simulink model "ThdRwLtStFwdBkwdIsPosChk"  (R2018b)
settings: Solver=FixedStepDiscrete  StartTime=0.0  StopTime=10.0  FixedStep=0.01  RelTol=1e-3
undefined symbols (not defined in the file or in its folder): KeSMSuThirdRwStFwdBkwdPosDelta_Val, KeSMSuThirdRwStFwdBkwdPosTolr_Val, KeSMSuVehicleModelConfig_Val
libraries: StIsPosChkLib x17, simulink x5
(part 1 of 2)
settings Model: Creator=sn2xws  LastModifiedBy=sn55gm
settings Model: ModifiedHistory=|
  | 2024.3.14
  | V2.3.0
  | Bug 813950 童锁Lock，Mode1_Easy Entry Mode 不应调用失败
  | 2024.7.5 V3.0.0 557模式流程V1.9
  | 2024.8.28 V3.0.1 Lug模式修改干涉判断成功的逻辑
  | 2024.9.6 V3.0.2 新增Md56，注释不用的模式
  | 2024.10.14 V3.0.3 新增Md57 Md58
  | 2024.10.28 V3.0.4 6s版本不选md12目标位置
  | 2024.11.11 V3.0.5 vip 判断成功不看三排
  | 2024.12.24 V3.0.6 CR 960542 7S智享退出模式左右同时调用时，三排座椅前后使用逻辑变更
  | 2025.2.19 V3.8.0 Bug 991386 Md1 三排占座时未移动且报了成功
  | 25.7.1 V3.13.0 新增Md61 Md62
  | 25.7.17 V3.13.1 BUG 1089114
  | 25.8.12 V3.13.2 BUG 1109205
settings DataIOCC: SaveFormat=StructureWithTime
settings OptimizationCC: DefaultParameterBehavior=Inlined  EnhancedBackFolding=on  PassReuseOutputArgsAs=Individual arguments  ZeroExternalMemoryAtStartup=off  ZeroInternalMemoryAtStartup=off  OptimizeBlockOrder=speed  DifferentSizesBufferReuse=on  OptimizationCustomize=off
settings DebuggingCC: ParameterTunabilityLossMsg=error
settings ModelReferenceCC: ModelReferenceNumInstancesAllowed=Single
settings SFSimCC: MATLABDynamicMemAlloc=off
settings RTWCC: SystemTargetFile=autosar.tlc  GenCodeOnly=on  TemplateMakefile=ert_default_tmf  Description=AUTOSAR  GenerateReport=on  IncludeHyperlinkInReport=on  LaunchReport=on  GenerateTraceInfo=on  GenerateTraceReport=on  GenerateTraceReportSl=on  GenerateTraceReportSf=on  GenerateTraceReportEml=on
settings CodeAppCC: ForceParamTrailComments=on  IgnoreCustomStorageClasses=off  OperatorAnnotations=on  SimulinkDataObjDesc=on  SFDataObjDesc=on  InsertBlockDesc=on
settings STFCustomTargetCC: TargetLangStandard=C99 (ISO)  MultiwordLength=256  ParMdlRefBuildCompliant=on  CompOptLevelCompliant=on  IncludeMdlTerminateFcn=off  CombineOutputUpdateFcns=on  SuppressErrorStatus=on  ERTCustomFileBanners=on  SupportNonFinite=off  SupportComplex=off  SupportContinuousTime=off  SupportNonInlinedSFcns=off  RemoveResetFunc=on  MATLABClassNameForMDSCustomization=Simulink.SoftwareTarget.ERTCustomization  AutosarCompliant=on  UseToolchainInfoCompliant=on  LookupTableObjectStructAxisOrder=2,1,3,4,...  LUTObjectStructOrderEvenSpacing=Size,Table,Breakpoints  SystemTargetFile=autosar.tlc
settings ERTTargetCC: TargetLangStandard=C99 (ISO)  ConcurrentExecutionCompliant=off  IncludeMdlTerminateFcn=off  SuppressErrorStatus=on  SupportNonFinite=off  SupportComplex=off  ModelStepFunctionPrototypeControlCompliant=off  CPPClassGenCompliant=off  AutosarCompliant=on  LookupTableObjectStructAxisOrder=2,1,3,4,...  LUTObjectStructOrderEvenSpacing=Size,Table,Breakpoints  InlinedParameterPlacement=NonHierarchical  ERTCustomFileTemplate=example_file_process.tlc  ERTFilePackagingFormat=Compact

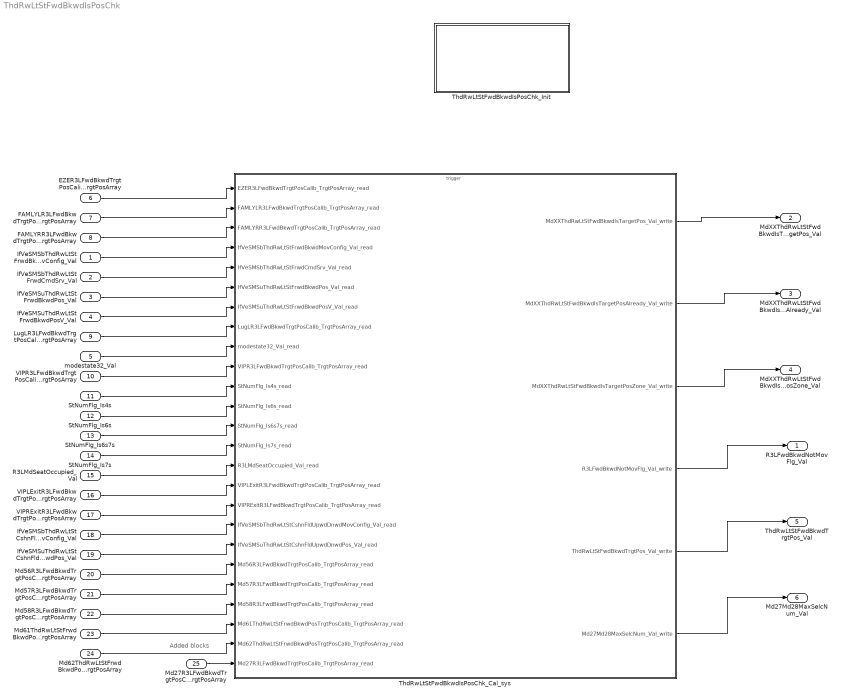
== system ThdRwLtStFwdBkwdIsPosChk ==
  note: Added blocks
  IfVeSMSbThdRwLtStFrwdBkwdMovConfig_Val : Inport  OutDataTypeStr=boolean  PortDimensions=1
  IfVeSMSbThdRwLtStFrwdCmdSrv_Val : Inport  Port=2  OutDataTypeStr=boolean  PortDimensions=1
  IfVeSMSuThdRwLtStFrwdBkwdPos_Val : Inport  Port=3  OutDataTypeStr=uint16  PortDimensions=1
  IfVeSMSuThdRwLtStFrwdBkwdPosV_Val : Inport  Port=4  OutDataTypeStr=boolean  PortDimensions=1
  modestate32_Val : Inport  Port=5  OutDataTypeStr=uint32  PortDimensions=1
  EZER3LFwdBkwdTrgtPosCalib_TrgtPosArray : Inport  Description=|  Port=6  OutDataTypeStr=uint16  PortDimensions=3
      | 0:Pos
      | 1:Max
      | 2:Min
  FAMLYLR3LFwdBkwdTrgtPosCalib_TrgtPosArray : Inport  Description=|  Port=7  OutDataTypeStr=uint16  PortDimensions=3
      | 0:Pos
      | 1:Max
      | 2:Min
  FAMLYRR3LFwdBkwdTrgtPosCalib_TrgtPosArray : Inport  Description=|  Port=8  OutDataTypeStr=uint16  PortDimensions=3
      | 0:Pos
      | 1:Max
      | 2:Min
  LugLR3LFwdBkwdTrgtPosCalib_TrgtPosArray : Inport  Description=|  Port=9  OutDataTypeStr=uint16  PortDimensions=3
      | 0:Pos
      | 1:Max
      | 2:Min
  VIPR3LFwdBkwdTrgtPosCalib_TrgtPosArray : Inport  Description=|  Port=10  OutDataTypeStr=uint16  PortDimensions=3
      | 0:Pos
      | 1:Max
      | 2:Min
  StNumFlg_Is4s : Inport  Port=11  OutDataTypeStr=boolean  PortDimensions=1
  StNumFlg_Is6s : Inport  Port=12  OutDataTypeStr=boolean  PortDimensions=1
  StNumFlg_Is6s7s : Inport  Port=13  OutDataTypeStr=boolean  PortDimensions=1
  StNumFlg_Is7s : Inport  Port=14  OutDataTypeStr=boolean  PortDimensions=1
  R3LMdSeatOccupied_Val : Inport  Port=15  OutDataTypeStr=boolean  PortDimensions=1
  VIPLExitR3LFwdBkwdTrgtPosCalib_TrgtPosArray : Inport  Description=|  Port=16  OutDataTypeStr=uint16  PortDimensions=3
      | 0:Pos
      | 1:Max
      | 2:Min
  VIPRExitR3LFwdBkwdTrgtPosCalib_TrgtPosArray : Inport  Description=|  Port=17  OutDataTypeStr=uint16  PortDimensions=3
      | 0:Pos
      | 1:Max
      | 2:Min
  IfVeSMSbThdRwLtStCshnFldUpwdDnwdMovConfig_Val : Inport  Port=18  OutDataTypeStr=boolean  PortDimensions=1
  IfVeSMSuThdRwLtStCshnFldUpwdDnwdPos_Val : Inport  Port=19  OutDataTypeStr=uint16  PortDimensions=1
  Md56R3LFwdBkwdTrgtPosCalib_TrgtPosArray : Inport  Description=|  Port=20  OutDataTypeStr=uint16  PortDimensions=3
      | 0:Pos
      | 1:Max
      | 2:Min
  Md57R3LFwdBkwdTrgtPosCalib_TrgtPosArray : Inport  Description=|  Port=21  OutDataTypeStr=uint16  PortDimensions=3
      | 0:Pos
      | 1:Max
      | 2:Min
  Md58R3LFwdBkwdTrgtPosCalib_TrgtPosArray : Inport  Description=|  Port=22  OutDataTypeStr=uint16  PortDimensions=3
      | 0:Pos
      | 1:Max
      | 2:Min
  Md61ThdRwLtStFrwdBkwdPosTrgtPosCalib_TrgtPosArray : Inport  Description=|  Port=23  OutDataTypeStr=uint16  PortDimensions=3
      | 0:Pos
      | 1:Max
      | 2:Min
  Md62ThdRwLtStFrwdBkwdPosTrgtPosCalib_TrgtPosArray : Inport  Description=|  Port=24  OutDataTypeStr=uint16  PortDimensions=3
      | 0:Pos
      | 1:Max
      | 2:Min
  Md27R3LFwdBkwdTrgtPosCalib_TrgtPosArray : Inport  Description=|  Port=25  OutDataTypeStr=uint16  PortDimensions=3
      | 0:Pos
      | 1:Max
      | 2:Min
  ThdRwLtStFwdBkwdIsPosChk_Cal_sys : Subsystem
  ThdRwLtStFwdBkwdIsPosChk_Init : Subsystem
  R3LFwdBkwdNotMovFlg_Val : Outport  OutDataTypeStr=boolean  PortDimensions=1
  MdXXThdRwLtStFwdBkwdIsTargetPos_Val : Outport  Port=2  OutDataTypeStr=uint32  PortDimensions=1
  MdXXThdRwLtStFwdBkwdIsTargetPosAlready_Val : Outport  Port=3  OutDataTypeStr=uint32  PortDimensions=1
  MdXXThdRwLtStFwdBkwdIsTargetPosZone_Val : Outport  Port=4  OutDataTypeStr=uint32  PortDimensions=1
  ThdRwLtStFwdBkwdTrgtPos_Val : Outport  Port=5  OutDataTypeStr=uint16  PortDimensions=1
  Md27Md28MaxSelcNum_Val : Outport  Port=6  OutDataTypeStr=uint8  PortDimensions=1
  wires:
  ThdRwLtStFwdBkwdIsPosChk_Cal_sys/1(MdXXThdRwLtStFwdBkwdIsTargetPos_Val_write) -> MdXXThdRwLtStFwdBkwdIsTargetPos_Val/1
  ThdRwLtStFwdBkwdIsPosChk_Cal_sys/2(MdXXThdRwLtStFwdBkwdIsTargetPosAlready_Val_write) -> MdXXThdRwLtStFwdBkwdIsTargetPosAlready_Val/1
  ThdRwLtStFwdBkwdIsPosChk_Cal_sys/3(MdXXThdRwLtStFwdBkwdIsTargetPosZone_Val_write) -> MdXXThdRwLtStFwdBkwdIsTargetPosZone_Val/1
  ThdRwLtStFwdBkwdIsPosChk_Cal_sys/4(R3LFwdBkwdNotMovFlg_Val_write) -> R3LFwdBkwdNotMovFlg_Val/1
  ThdRwLtStFwdBkwdIsPosChk_Cal_sys/5(ThdRwLtStFwdBkwdTrgtPos_Val_write) -> ThdRwLtStFwdBkwdTrgtPos_Val/1
  EZER3LFwdBkwdTrgtPosCalib_TrgtPosArray/1 -> ThdRwLtStFwdBkwdIsPosChk_Cal_sys/1(EZER3LFwdBkwdTrgtPosCalib_TrgtPosArray_read)
  FAMLYLR3LFwdBkwdTrgtPosCalib_TrgtPosArray/1 -> ThdRwLtStFwdBkwdIsPosChk_Cal_sys/2(FAMLYLR3LFwdBkwdTrgtPosCalib_TrgtPosArray_read)
  FAMLYRR3LFwdBkwdTrgtPosCalib_TrgtPosArray/1 -> ThdRwLtStFwdBkwdIsPosChk_Cal_sys/3(FAMLYRR3LFwdBkwdTrgtPosCalib_TrgtPosArray_read)
  IfVeSMSbThdRwLtStFrwdBkwdMovConfig_Val/1 -> ThdRwLtStFwdBkwdIsPosChk_Cal_sys/4(IfVeSMSbThdRwLtStFrwdBkwdMovConfig_Val_read)
  IfVeSMSbThdRwLtStFrwdCmdSrv_Val/1 -> ThdRwLtStFwdBkwdIsPosChk_Cal_sys/5(IfVeSMSbThdRwLtStFrwdCmdSrv_Val_read)
  IfVeSMSuThdRwLtStFrwdBkwdPos_Val/1 -> ThdRwLtStFwdBkwdIsPosChk_Cal_sys/6(IfVeSMSuThdRwLtStFrwdBkwdPos_Val_read)
  IfVeSMSuThdRwLtStFrwdBkwdPosV_Val/1 -> ThdRwLtStFwdBkwdIsPosChk_Cal_sys/7(IfVeSMSuThdRwLtStFrwdBkwdPosV_Val_read)
  LugLR3LFwdBkwdTrgtPosCalib_TrgtPosArray/1 -> ThdRwLtStFwdBkwdIsPosChk_Cal_sys/8(LugLR3LFwdBkwdTrgtPosCalib_TrgtPosArray_read)
  modestate32_Val/1 -> ThdRwLtStFwdBkwdIsPosChk_Cal_sys/9(modestate32_Val_read)
  VIPR3LFwdBkwdTrgtPosCalib_TrgtPosArray/1 -> ThdRwLtStFwdBkwdIsPosChk_Cal_sys/10(VIPR3LFwdBkwdTrgtPosCalib_TrgtPosArray_read)
  StNumFlg_Is4s/1 -> ThdRwLtStFwdBkwdIsPosChk_Cal_sys/11(StNumFlg_Is4s_read)
  StNumFlg_Is6s/1 -> ThdRwLtStFwdBkwdIsPosChk_Cal_sys/12(StNumFlg_Is6s_read)
  StNumFlg_Is6s7s/1 -> ThdRwLtStFwdBkwdIsPosChk_Cal_sys/13(StNumFlg_Is6s7s_read)
  StNumFlg_Is7s/1 -> ThdRwLtStFwdBkwdIsPosChk_Cal_sys/14(StNumFlg_Is7s_read)
  R3LMdSeatOccupied_Val/1 -> ThdRwLtStFwdBkwdIsPosChk_Cal_sys/15(R3LMdSeatOccupied_Val_read)
  VIPLExitR3LFwdBkwdTrgtPosCalib_TrgtPosArray/1 -> ThdRwLtStFwdBkwdIsPosChk_Cal_sys/16(VIPLExitR3LFwdBkwdTrgtPosCalib_TrgtPosArray_read)
  VIPRExitR3LFwdBkwdTrgtPosCalib_TrgtPosArray/1 -> ThdRwLtStFwdBkwdIsPosChk_Cal_sys/17(VIPRExitR3LFwdBkwdTrgtPosCalib_TrgtPosArray_read)
  IfVeSMSbThdRwLtStCshnFldUpwdDnwdMovConfig_Val/1 -> ThdRwLtStFwdBkwdIsPosChk_Cal_sys/18(IfVeSMSbThdRwLtStCshnFldUpwdDnwdMovConfig_Val_read)
  IfVeSMSuThdRwLtStCshnFldUpwdDnwdPos_Val/1 -> ThdRwLtStFwdBkwdIsPosChk_Cal_sys/19(IfVeSMSuThdRwLtStCshnFldUpwdDnwdPos_Val_read)
  Md56R3LFwdBkwdTrgtPosCalib_TrgtPosArray/1 -> ThdRwLtStFwdBkwdIsPosChk_Cal_sys/20(Md56R3LFwdBkwdTrgtPosCalib_TrgtPosArray_read)
  Md57R3LFwdBkwdTrgtPosCalib_TrgtPosArray/1 -> ThdRwLtStFwdBkwdIsPosChk_Cal_sys/21(Md57R3LFwdBkwdTrgtPosCalib_TrgtPosArray_read)
  Md58R3LFwdBkwdTrgtPosCalib_TrgtPosArray/1 -> ThdRwLtStFwdBkwdIsPosChk_Cal_sys/22(Md58R3LFwdBkwdTrgtPosCalib_TrgtPosArray_read)
  ThdRwLtStFwdBkwdIsPosChk_Cal_sys/6(Md27Md28MaxSelcNum_Val_write) -> Md27Md28MaxSelcNum_Val/1
  Md61ThdRwLtStFrwdBkwdPosTrgtPosCalib_TrgtPosArray/1 -> ThdRwLtStFwdBkwdIsPosChk_Cal_sys/23(Md61ThdRwLtStFrwdBkwdPosTrgtPosCalib_TrgtPosArray_read)
  Md62ThdRwLtStFrwdBkwdPosTrgtPosCalib_TrgtPosArray/1 -> ThdRwLtStFwdBkwdIsPosChk_Cal_sys/24(Md62ThdRwLtStFrwdBkwdPosTrgtPosCalib_TrgtPosArray_read)
  Md27R3LFwdBkwdTrgtPosCalib_TrgtPosArray/1 -> ThdRwLtStFwdBkwdIsPosChk_Cal_sys/25(Md27R3LFwdBkwdTrgtPosCalib_TrgtPosArray_read)

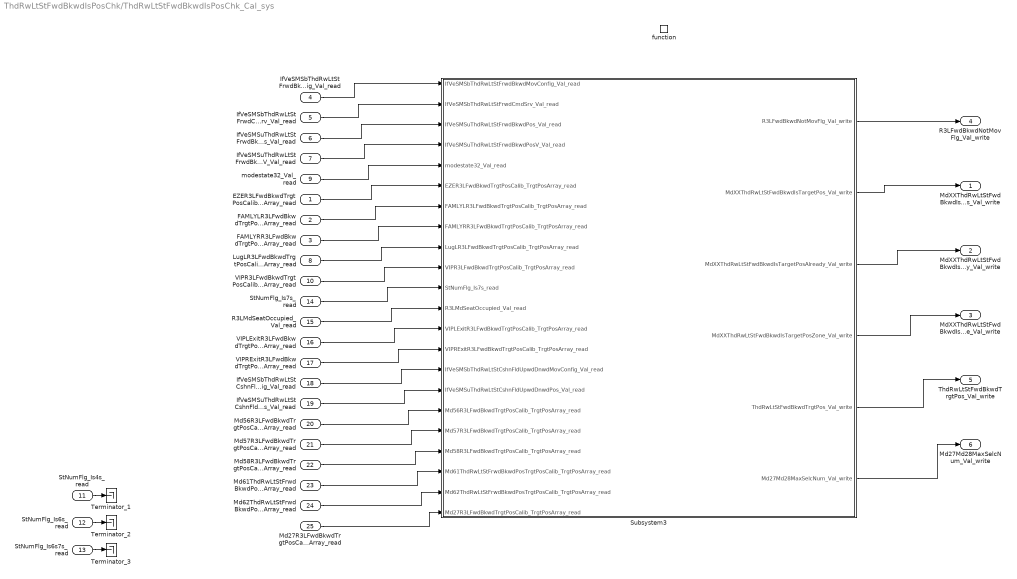
== system ThdRwLtStFwdBkwdIsPosChk/ThdRwLtStFwdBkwdIsPosChk_Cal_sys ==
  EZER3LFwdBkwdTrgtPosCalib_TrgtPosArray_read : Inport
  FAMLYLR3LFwdBkwdTrgtPosCalib_TrgtPosArray_read : Inport  Port=2
  FAMLYRR3LFwdBkwdTrgtPosCalib_TrgtPosArray_read : Inport  Port=3
  IfVeSMSbThdRwLtStFrwdBkwdMovConfig_Val_read : Inport  Port=4
  IfVeSMSbThdRwLtStFrwdCmdSrv_Val_read : Inport  Port=5
  IfVeSMSuThdRwLtStFrwdBkwdPos_Val_read : Inport  Port=6
  IfVeSMSuThdRwLtStFrwdBkwdPosV_Val_read : Inport  Port=7
  LugLR3LFwdBkwdTrgtPosCalib_TrgtPosArray_read : Inport  Port=8
  modestate32_Val_read : Inport  Port=9
  VIPR3LFwdBkwdTrgtPosCalib_TrgtPosArray_read : Inport  Port=10
  StNumFlg_Is4s_read : Inport  Port=11
  StNumFlg_Is6s_read : Inport  Port=12
  StNumFlg_Is6s7s_read : Inport  Port=13
  StNumFlg_Is7s_read : Inport  Port=14
  R3LMdSeatOccupied_Val_read : Inport  Port=15
  VIPLExitR3LFwdBkwdTrgtPosCalib_TrgtPosArray_read : Inport  Port=16
  VIPRExitR3LFwdBkwdTrgtPosCalib_TrgtPosArray_read : Inport  Port=17
  IfVeSMSbThdRwLtStCshnFldUpwdDnwdMovConfig_Val_read : Inport  Port=18
  IfVeSMSuThdRwLtStCshnFldUpwdDnwdPos_Val_read : Inport  Port=19
  Md56R3LFwdBkwdTrgtPosCalib_TrgtPosArray_read : Inport  Port=20
  Md57R3LFwdBkwdTrgtPosCalib_TrgtPosArray_read : Inport  Port=21
  Md58R3LFwdBkwdTrgtPosCalib_TrgtPosArray_read : Inport  Port=22
  Md61ThdRwLtStFrwdBkwdPosTrgtPosCalib_TrgtPosArray_read : Inport  Port=23
  Md62ThdRwLtStFrwdBkwdPosTrgtPosCalib_TrgtPosArray_read : Inport  Port=24
  Md27R3LFwdBkwdTrgtPosCalib_TrgtPosArray_read : Inport  Port=25
  function : TriggerPort  TriggerType=function-call  IsSimulinkFunction=on  FunctionName=ThdRwLtStFwdBkwdIsPosChk_Cal  VariantControl=(inherit)
  Subsystem3 : Subsystem
  Terminator_1 : Terminator
  Terminator_2 : Terminator
  Terminator_3 : Terminator
  MdXXThdRwLtStFwdBkwdIsTargetPos_Val_write : Outport
      settings: EnsureOutportIsVirtual=on
  MdXXThdRwLtStFwdBkwdIsTargetPosAlready_Val_write : Outport  Port=2
      settings: EnsureOutportIsVirtual=on
  MdXXThdRwLtStFwdBkwdIsTargetPosZone_Val_write : Outport  Port=3
      settings: EnsureOutportIsVirtual=on
  R3LFwdBkwdNotMovFlg_Val_write : Outport  Port=4
      settings: EnsureOutportIsVirtual=on
  ThdRwLtStFwdBkwdTrgtPos_Val_write : Outport  Port=5
      settings: EnsureOutportIsVirtual=on
  Md27Md28MaxSelcNum_Val_write : Outport  Port=6
      settings: EnsureOutportIsVirtual=on
  wires:
  Subsystem3/1(R3LFwdBkwdNotMovFlg_Val_write) -> R3LFwdBkwdNotMovFlg_Val_write/1
  Subsystem3/2(MdXXThdRwLtStFwdBkwdIsTargetPos_Val_write) -> MdXXThdRwLtStFwdBkwdIsTargetPos_Val_write/1
  Subsystem3/3(MdXXThdRwLtStFwdBkwdIsTargetPosAlready_Val_write) -> MdXXThdRwLtStFwdBkwdIsTargetPosAlready_Val_write/1
  Subsystem3/4(MdXXThdRwLtStFwdBkwdIsTargetPosZone_Val_write) -> MdXXThdRwLtStFwdBkwdIsTargetPosZone_Val_write/1
  Subsystem3/5(ThdRwLtStFwdBkwdTrgtPos_Val_write) -> ThdRwLtStFwdBkwdTrgtPos_Val_write/1
  IfVeSMSbThdRwLtStFrwdBkwdMovConfig_Val_read/1 -> Subsystem3/1(IfVeSMSbThdRwLtStFrwdBkwdMovConfig_Val_read)
  IfVeSMSbThdRwLtStFrwdCmdSrv_Val_read/1 -> Subsystem3/2(IfVeSMSbThdRwLtStFrwdCmdSrv_Val_read)
  IfVeSMSuThdRwLtStFrwdBkwdPos_Val_read/1 -> Subsystem3/3(IfVeSMSuThdRwLtStFrwdBkwdPos_Val_read)
  IfVeSMSuThdRwLtStFrwdBkwdPosV_Val_read/1 -> Subsystem3/4(IfVeSMSuThdRwLtStFrwdBkwdPosV_Val_read)
  modestate32_Val_read/1 -> Subsystem3/5(modestate32_Val_read)
  EZER3LFwdBkwdTrgtPosCalib_TrgtPosArray_read/1 -> Subsystem3/6(EZER3LFwdBkwdTrgtPosCalib_TrgtPosArray_read)
  FAMLYLR3LFwdBkwdTrgtPosCalib_TrgtPosArray_read/1 -> Subsystem3/7(FAMLYLR3LFwdBkwdTrgtPosCalib_TrgtPosArray_read)
  FAMLYRR3LFwdBkwdTrgtPosCalib_TrgtPosArray_read/1 -> Subsystem3/8(FAMLYRR3LFwdBkwdTrgtPosCalib_TrgtPosArray_read)
  LugLR3LFwdBkwdTrgtPosCalib_TrgtPosArray_read/1 -> Subsystem3/9(LugLR3LFwdBkwdTrgtPosCalib_TrgtPosArray_read)
  VIPR3LFwdBkwdTrgtPosCalib_TrgtPosArray_read/1 -> Subsystem3/10(VIPR3LFwdBkwdTrgtPosCalib_TrgtPosArray_read)
  StNumFlg_Is4s_read/1 -> Terminator_1/1
  StNumFlg_Is6s_read/1 -> Terminator_2/1
  StNumFlg_Is6s7s_read/1 -> Terminator_3/1
  StNumFlg_Is7s_read/1 -> Subsystem3/11(StNumFlg_Is7s_read)
  R3LMdSeatOccupied_Val_read/1 -> Subsystem3/12(R3LMdSeatOccupied_Val_read)
  VIPLExitR3LFwdBkwdTrgtPosCalib_TrgtPosArray_read/1 -> Subsystem3/13(VIPLExitR3LFwdBkwdTrgtPosCalib_TrgtPosArray_read)
  VIPRExitR3LFwdBkwdTrgtPosCalib_TrgtPosArray_read/1 -> Subsystem3/14(VIPRExitR3LFwdBkwdTrgtPosCalib_TrgtPosArray_read)
  IfVeSMSbThdRwLtStCshnFldUpwdDnwdMovConfig_Val_read/1 -> Subsystem3/15(IfVeSMSbThdRwLtStCshnFldUpwdDnwdMovConfig_Val_read)
  IfVeSMSuThdRwLtStCshnFldUpwdDnwdPos_Val_read/1 -> Subsystem3/16(IfVeSMSuThdRwLtStCshnFldUpwdDnwdPos_Val_read)
  Md56R3LFwdBkwdTrgtPosCalib_TrgtPosArray_read/1 -> Subsystem3/17(Md56R3LFwdBkwdTrgtPosCalib_TrgtPosArray_read)
  Md57R3LFwdBkwdTrgtPosCalib_TrgtPosArray_read/1 -> Subsystem3/18(Md57R3LFwdBkwdTrgtPosCalib_TrgtPosArray_read)
  Md58R3LFwdBkwdTrgtPosCalib_TrgtPosArray_read/1 -> Subsystem3/19(Md58R3LFwdBkwdTrgtPosCalib_TrgtPosArray_read)
  Subsystem3/6(Md27Md28MaxSelcNum_Val_write) -> Md27Md28MaxSelcNum_Val_write/1
  Md61ThdRwLtStFrwdBkwdPosTrgtPosCalib_TrgtPosArray_read/1 -> Subsystem3/20(Md61ThdRwLtStFrwdBkwdPosTrgtPosCalib_TrgtPosArray_read)
  Md62ThdRwLtStFrwdBkwdPosTrgtPosCalib_TrgtPosArray_read/1 -> Subsystem3/21(Md62ThdRwLtStFrwdBkwdPosTrgtPosCalib_TrgtPosArray_read)
  ? -> ?
  Md27R3LFwdBkwdTrgtPosCalib_TrgtPosArray_read/1 -> Subsystem3/22(Md27R3LFwdBkwdTrgtPosCalib_TrgtPosArray_read)

== system ThdRwLtStFwdBkwdIsPosChk/ThdRwLtStFwdBkwdIsPosChk_Init ==
  note: Added blocks
  note: Added blocks
  note: Added blocks
  Event Listener : EventListener  EventName=reset
  PA_KeSMSuThirdRwStFwdBkwdPosDelta_Val : Constant  Value=KeSMSuThirdRwStFwdBkwdPosDelta_Val
  PA_KeSMSuThirdRwStFwdBkwdPosTolr_Val : Constant  Value=KeSMSuThirdRwStFwdBkwdPosTolr_Val
  PA_KeSMSuVehicleModelConfig_Val : Constant  Value=KeSMSuVehicleModelConfig_Val
  Terminator_1 : Terminator
  Terminator_2 : Terminator
  Terminator_3 : Terminator
  wires:
  PA_KeSMSuThirdRwStFwdBkwdPosDelta_Val/1 -> Terminator_1/1
  PA_KeSMSuThirdRwStFwdBkwdPosTolr_Val/1 -> Terminator_2/1
  PA_KeSMSuVehicleModelConfig_Val/1 -> Terminator_3/1

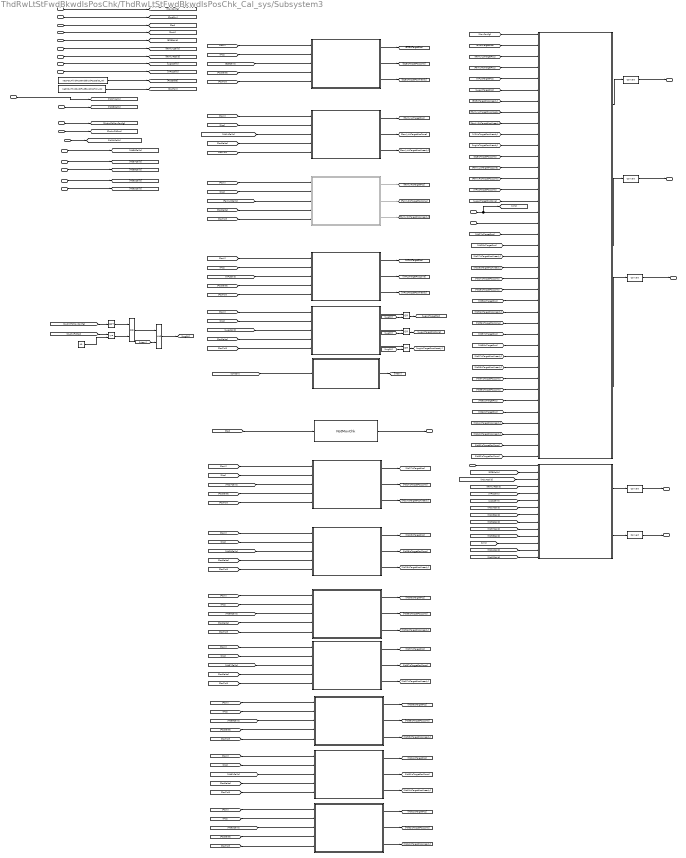
== system ThdRwLtStFwdBkwdIsPosChk/ThdRwLtStFwdBkwdIsPosChk_Cal_sys/Subsystem3 ==
  note: 增加逻辑Lug模式非干涉但是到最前了算成功
  IfVeSMSbThdRwLtStFrwdBkwdMovConfig_Val_read : Inport
  IfVeSMSbThdRwLtStFrwdCmdSrv_Val_read : Inport  Port=2
  IfVeSMSuThdRwLtStFrwdBkwdPos_Val_read : Inport  Port=3
  IfVeSMSuThdRwLtStFrwdBkwdPosV_Val_read : Inport  Port=4
  modestate32_Val_read : Inport  Port=5
  EZER3LFwdBkwdTrgtPosCalib_TrgtPosArray_read : Inport  Port=6
  FAMLYLR3LFwdBkwdTrgtPosCalib_TrgtPosArray_read : Inport  Port=7
  FAMLYRR3LFwdBkwdTrgtPosCalib_TrgtPosArray_read : Inport  Port=8
  LugLR3LFwdBkwdTrgtPosCalib_TrgtPosArray_read : Inport  Port=9
  VIPR3LFwdBkwdTrgtPosCalib_TrgtPosArray_read : Inport  Port=10
  StNumFlg_Is7s_read : Inport  Port=11
  R3LMdSeatOccupied_Val_read : Inport  Port=12
  VIPLExitR3LFwdBkwdTrgtPosCalib_TrgtPosArray_read : Inport  Port=13
  VIPRExitR3LFwdBkwdTrgtPosCalib_TrgtPosArray_read : Inport  Port=14
  IfVeSMSbThdRwLtStCshnFldUpwdDnwdMovConfig_Val_read : Inport  Port=15
  IfVeSMSuThdRwLtStCshnFldUpwdDnwdPos_Val_read : Inport  Port=16
  Md56R3LFwdBkwdTrgtPosCalib_TrgtPosArray_read : Inport  Port=17
  Md57R3LFwdBkwdTrgtPosCalib_TrgtPosArray_read : Inport  Port=18
  Md58R3LFwdBkwdTrgtPosCalib_TrgtPosArray_read : Inport  Port=19
  Md61ThdRwLtStFrwdBkwdPosTrgtPosCalib_TrgtPosArray_read : Inport  Port=20
  Md62ThdRwLtStFrwdBkwdPosTrgtPosCalib_TrgtPosArray_read : Inport  Port=21
  Md27R3LFwdBkwdTrgtPosCalib_TrgtPosArray_read : Inport  Port=22
  Constant : Constant  Value=40  OutDataTypeStr=uint16
  Data Type Conversion{,1..4} (5 alike) : DataTypeConversion
  Logical Operator{,1,4..5} (4 alike) : Logic  Operator=OR  AllPortsSameDT=off  OutDataTypeStr=boolean
  Logical Operator2 : Logic  Operator=NOT  AllPortsSameDT=off  OutDataTypeStr=boolean
  Logical Operator3 : Logic  AllPortsSameDT=off  OutDataTypeStr=boolean
  NotMovChk : StIsPosChkLib/NotMovChk  SystemSampleTime=-1
  PA_KeSMSuThirdRwStFwdBkwdPosDelta_Val : Constant  Value=KeSMSuThirdRwStFwdBkwdPosDelta_Val
  PA_KeSMSuThirdRwStFwdBkwdPosTolr_Val : Constant  Value=KeSMSuThirdRwStFwdBkwdPosTolr_Val
  Relational Operator : RelationalOperator  Operator=<=  OutDataTypeStr=boolean  RndMeth=Simplest
  Subsystem : Subsystem
  Subsystem1 : Subsystem
  Subsystem10 : Subsystem
  Subsystem11 : Subsystem
  Subsystem12 : Subsystem
  Subsystem13 : Subsystem
  Subsystem14 : Subsystem
  Subsystem2 : Subsystem
  Subsystem3 : Subsystem
  Subsystem4 : Subsystem
  Subsystem5 : Subsystem  Commented=on
  Subsystem6 : Subsystem
  Subsystem7 : Subsystem
  Subsystem8 : Subsystem
  Subsystem9 : Subsystem
  R3LFwdBkwdNotMovFlg_Val_write : Outport
      settings: EnsureOutportIsVirtual=on
  MdXXThdRwLtStFwdBkwdIsTargetPos_Val_write : Outport  Port=2
      settings: EnsureOutportIsVirtual=on
  MdXXThdRwLtStFwdBkwdIsTargetPosAlready_Val_write : Outport  Port=3
      settings: EnsureOutportIsVirtual=on
  MdXXThdRwLtStFwdBkwdIsTargetPosZone_Val_write : Outport  Port=4
      settings: EnsureOutportIsVirtual=on
  ThdRwLtStFwdBkwdTrgtPos_Val_write : Outport  Port=5
      settings: EnsureOutportIsVirtual=on
  Md27Md28MaxSelcNum_Val_write : Outport  Port=6
      settings: EnsureOutportIsVirtual=on
  wires:
  [PosV] -> Subsystem5/1(PosV)
  Subsystem1/3(IsTargetPosZone) -> Data Type Conversion3/1
  [PosTolr] -> Subsystem5/5(Tolr)
  IfVeSMSuThdRwLtStFrwdBkwdPos_Val_read/1 -> [Pos]
  Data Type Conversion3/1 -> MdXXThdRwLtStFwdBkwdIsTargetPosZone_Val_write/1
  [VIPLCalib] -> Subsystem6/3(CalibArray)
  Subsystem/1(TrgtPos) -> Data Type Conversion/1
  IfVeSMSuThdRwLtStFrwdBkwdPosV_Val_read/1 -> [PosV]
  FAMLYRR3LFwdBkwdTrgtPosCalib_TrgtPosArray_read/1 -> [FamlyRCalib]
  [Pos] -> Subsystem3/2(Pos)
  [LugLIsTargetPosAlready] -> Subsystem1/11(INTMLIsTargetPosAlready)
  EZER3LFwdBkwdTrgtPosCalib_TrgtPosArray_read/1 -> [EZECalib]
  [EZEIsTargetPos] -> Subsystem1/2(EZEIsTargetPos)
  PA_KeSMSuThirdRwStFwdBkwdPosDelta_Val/1 -> [PosDelta]
  IfVeSMSbThdRwLtStFrwdCmdSrv_Val_read/1 -> [CmdSrv]
  [VIPLIsTargetPosZone] -> Subsystem1/15(VIPLIsTargetPosZone)
  PA_KeSMSuThirdRwStFwdBkwdPosTolr_Val/1 -> [PosTolr]
  [PosTolr] -> Subsystem3/5(Tolr)
  [LugLIsTargetPos] -> Subsystem1/6(INTMLIsTargetPos)
  Subsystem4/1(IsPos) -> [EZEIsTargetPos]
  VIPR3LFwdBkwdTrgtPosCalib_TrgtPosArray_read/1 -> [VIPLCalib]
  LugLR3LFwdBkwdTrgtPosCalib_TrgtPosArray_read/1 -> [LugLCalib]
  [FamlyRCalib] -> Subsystem5/3(CalibArray)
  [PosDelta] -> Subsystem6/4(Delta)
  [PosDelta] -> Subsystem5/4(Delta)
  [PosV] -> Subsystem4/1(PosV)
  [FamlyLIsTargetPos] -> Subsystem1/3(FamlyLIsTargetPos)
  [FamlyRIsTargetPosZone] -> Subsystem1/14(FamlyRIsTargetPosZone)
  Subsystem6/2(IsPosZone) -> [VIPLIsTargetPosZone]
  [PosDelta] -> Subsystem4/4(Delta)
  [EZEIsTargetPosAlready] -> Subsystem1/7(EZEIsTargetPosAlready)
  NotMovChk/1 -> R3LFwdBkwdNotMovFlg_Val_write/1
  [PosV] -> Subsystem3/1(PosV)
  Data Type Conversion2/1 -> MdXXThdRwLtStFwdBkwdIsTargetPosAlready_Val_write/1
  [FamlyLIsTargetPosZone] -> Subsystem1/13(FamlyLIsTargetPosZone)
  [Pos] -> Subsystem6/2(Pos)
  Subsystem1/2(IsTargetPosAlready) -> Data Type Conversion2/1
  Subsystem3/2(IsPosZone) -> [FamlyLIsTargetPosZone]
  FAMLYLR3LFwdBkwdTrgtPosCalib_TrgtPosArray_read/1 -> [FamlyLCalib]
  [LugLCalib] -> Subsystem/6(LugLCalib)
  [FamlyRIsTargetPosAlready] -> Subsystem1/9(FamlyRIsTargetPosAlready)
  Subsystem4/3(IsPosAlready) -> [EZEIsTargetPosAlready]
  [Pos] -> NotMovChk/1
  [Pos] -> Subsystem4/2(Pos)
  [PosTolr] -> Subsystem4/5(Tolr)
  Subsystem3/3(IsPosAlready) -> [FamlyLIsTargetPosAlready]
  [PosTolr] -> Subsystem6/5(Tolr)
  Subsystem4/2(IsPosZone) -> [EZEIsTargetPosZone]
  Subsystem5/1(IsPos) -> [FamlyRIsTargetPos]
  Subsystem5/3(IsPosAlready) -> [FamlyRIsTargetPosAlready]
  Subsystem1/1(IsTargetPos) -> Data Type Conversion1/1
  [PosV] -> Subsystem6/1(PosV)
  Subsystem6/3(IsPosAlready) -> [VIPLIsTargetPosAlready]
  [VIPLIsTargetPosAlready] -> Subsystem1/10(VIPLIsTargetPosAlready)
  [EZECalib] -> Subsystem4/3(CalibArray)
  [LugLIsTargetPosZone] -> Subsystem1/16(INTMLIsTargetPosZone)
  [VIPLIsTargetPos] -> Subsystem1/5(VIPLIsTargetPos)
  [Md14Calib] -> Subsystem/3(Md14Calib)
  [FamlyRIsTargetPos] -> Subsystem1/4(FamlyRIsTargetPos)
  Subsystem6/1(IsPos) -> [VIPLIsTargetPos]
  [MovConfig] -> Subsystem1/1(MovConfig)
  [EZECalib] -> Subsystem/2(EZECalib)
  Subsystem5/2(IsPosZone) -> [FamlyRIsTargetPosZone]
  [Pos] -> Subsystem5/2(Pos)
  IfVeSMSbThdRwLtStFrwdBkwdMovConfig_Val_read/1 -> [MovConfig]
  [VIPLCalib] -> Subsystem/5(VIPLCalib)
  [PosDelta] -> Subsystem3/4(Delta)
  [FamlyRCalib] -> Subsystem/4(FamlyRCalib)
  modestate32_Val_read/1 -> Subsystem/1(modestate32_Val_read)
  [FamlyLIsTargetPosAlready] -> Subsystem1/8(FamlyLIsTargetPosAlready)
  Data Type Conversion/1 -> ThdRwLtStFwdBkwdTrgtPos_Val_write/1
  Subsystem3/1(IsPos) -> [FamlyLIsTargetPos]
  [CmdSrv] -> Subsystem2/1(CmdSrv)
  [EZEIsTargetPosZone] -> Subsystem1/12(EZEIsTargetPosZone)
  Data Type Conversion1/1 -> MdXXThdRwLtStFwdBkwdIsTargetPos_Val_write/1
  StNumFlg_Is7s_read/1 -> [is7s], Subsystem1/17(StNumFlg_Is7s_read)
  [PosV] -> Subsystem7/1(PosV)
  [PosTolr] -> Subsystem7/5(Tolr)
  [Pos] -> Subsystem7/2(Pos)
  [PosDelta] -> Subsystem7/4(Delta)
  [LugLCalib] -> Subsystem7/3(CalibArray)
  Subsystem2/1(IsTargetPos) -> [interv]
  Logical Operator1/1 -> [LugLIsTargetPosZone]
  [LugOK] -> Logical Operator1/2
  Subsystem7/2(IsPosZone) -> Logical Operator1/1
  R3LMdSeatOccupied_Val_read/1 -> Subsystem1/18(R3LMdSeatOccupied_Val_read)
  VIPRExitR3LFwdBkwdTrgtPosCalib_TrgtPosArray_read/1 -> [Md28Calib]
  Subsystem8/1(IsPos) -> [Md27IsTargetPos]
  Subsystem8/3(IsPosAlready) -> [Md27IsTargetPosAlready]
  [PosV] -> Subsystem8/1(PosV)
  [PosTolr] -> Subsystem8/5(Tolr)
  [Pos] -> Subsystem8/2(Pos)
  Subsystem8/2(IsPosZone) -> [Md27IsTargetPosZone]
  [PosDelta] -> Subsystem8/4(Delta)
  [Md27Calib] -> Subsystem8/3(CalibArray)
  [Md28Calib] -> Subsystem9/3(CalibArray)
  [PosDelta] -> Subsystem9/4(Delta)
  [Pos] -> Subsystem9/2(Pos)
  [PosTolr] -> Subsystem9/5(Tolr)
  [PosV] -> Subsystem9/1(PosV)
  Subsystem9/2(IsPosZone) -> [Md28IsTargetPosZone]
  Subsystem9/3(IsPosAlready) -> [Md28IsTargetPosAlready]
  Subsystem9/1(IsPos) -> [Md28IsTargetPos]
  [Md27Calib] -> Subsystem/7(Md27Calib)
  [Md28Calib] -> Subsystem/8(Md28Calib)
  [Md27IsTargetPos] -> Subsystem1/19(Md27IsTargetPos)
  [Md27IsTargetPosZone] -> Subsystem1/23(Md27IsTargetPosZone)
  [Md27IsTargetPosAlready] -> Subsystem1/21(Md27IsTargetPosAlready)
  [Md28IsTargetPos] -> Subsystem1/20(Md28IsTargetPos)
  [Md28IsTargetPosZone] -> Subsystem1/24(Md28IsTargetPosZone)
  [Md28IsTargetPosAlready] -> Subsystem1/22(Md28IsTargetPosAlready)
  IfVeSMSbThdRwLtStCshnFldUpwdDnwdMovConfig_Val_read/1 -> [CushnFldMovConfig]
  IfVeSMSuThdRwLtStCshnFldUpwdDnwdPos_Val_read/1 -> [CushnFldPos]
  [CushnFldMovConfig] -> Logical Operator2/1
  Logical Operator2/1 -> Logical Operator/1
  [CushnFldPos] -> Relational Operator/1
  Relational Operator/1 -> Logical Operator/2
  Constant/1 -> Relational Operator/2
  Logical Operator/1 -> Logical Operator3/1
  [interv] -> Logical Operator3/2
  Logical Operator3/1 -> [LugOK]
  Logical Operator4/1 -> [LugLIsTargetPos]
  Subsystem7/1(IsPos) -> Logical Operator4/1
  [LugOK] -> Logical Operator4/2
  Logical Operator5/1 -> [LugLIsTargetPosAlready]
  [LugOK] -> Logical Operator5/2
  Subsystem7/3(IsPosAlready) -> Logical Operator5/1
  Md56R3LFwdBkwdTrgtPosCalib_TrgtPosArray_read/1 -> [Md56Calib]
  Subsystem10/1(IsPos) -> [Md56IsTargetPos]
  Subsystem10/3(IsPosAlready) -> [Md56IsTargetPosAlready]
  Subsystem10/2(IsPosZone) -> [Md56IsTargetPosZone]
  [PosV] -> Subsystem10/1(PosV)
  [PosTolr] -> Subsystem10/5(Tolr)
  [Pos] -> Subsystem10/2(Pos)
  [PosDelta] -> Subsystem10/4(Delta)
  [Md56Calib] -> Subsystem10/3(CalibArray)
  [Md56Calib] -> Subsystem/9(Md56Calib)
  [Md56IsTargetPos] -> Subsystem1/25(Md56IsTargetPos)
  [Md56IsTargetPosZone] -> Subsystem1/27(Md56IsTargetPosZone)
  [Md56IsTargetPosAlready] -> Subsystem1/26(Md56IsTargetPosAlready)
  Md58R3LFwdBkwdTrgtPosCalib_TrgtPosArray_read/1 -> [Md58Calib]
  Md57R3LFwdBkwdTrgtPosCalib_TrgtPosArray_read/1 -> [Md57Calib]
  [Md57Calib] -> Subsystem11/3(CalibArray)
  [PosDelta] -> Subsystem11/4(Delta)
  [Pos] -> Subsystem11/2(Pos)
  [PosTolr] -> Subsystem11/5(Tolr)
  [PosV] -> Subsystem11/1(PosV)
  Subsystem11/2(IsPosZone) -> [Md57IsTargetPosZone]
  Subsystem11/3(IsPosAlready) -> [Md57IsTargetPosAlready]
  Subsystem11/1(IsPos) -> [Md57IsTargetPos]
  Subsystem12/1(IsPos) -> [Md58IsTargetPos]
  Subsystem12/3(IsPosAlready) -> [Md58IsTargetPosAlready]
  Subsystem12/2(IsPosZone) -> [Md58IsTargetPosZone]
  [PosV] -> Subsystem12/1(PosV)
  [PosTolr] -> Subsystem12/5(Tolr)
  [Pos] -> Subsystem12/2(Pos)
  [PosDelta] -> Subsystem12/4(Delta)
  [Md58Calib] -> Subsystem12/3(CalibArray)
  [Md58Calib] -> Subsystem/11(Md58Calib)
  [Md57Calib] -> Subsystem/10(Md76Calib)
  [Md58IsTargetPos] -> Subsystem1/29(Md58IsTargetPos)
  [Md57IsTargetPos] -> Subsystem1/28(Md57IsTargetPos)
  [Md57IsTargetPosZone] -> Subsystem1/32(Md57IsTargetPosZone)
  [Md58IsTargetPosZone] -> Subsystem1/33(Md58IsTargetPosZone)
  [Md57IsTargetPosAlready] -> Subsystem1/30(Md57IsTargetPosAlready)
  [Md58IsTargetPosAlready] -> Subsystem1/31(Md58IsTargetPosAlready)
  [is7s] -> Subsystem/12(is7s)
  Subsystem/2(Md27Md28MaxSelcNum_Val_write) -> Data Type Conversion4/1
  Data Type Conversion4/1 -> Md27Md28MaxSelcNum_Val_write/1
  Md61ThdRwLtStFrwdBkwdPosTrgtPosCalib_TrgtPosArray_read/1 -> [Md61Calib]
  Md62ThdRwLtStFrwdBkwdPosTrgtPosCalib_TrgtPosArray_read/1 -> [Md62Calib]
  [Md61Calib] -> Subsystem13/3(CalibArray)
  [PosDelta] -> Subsystem13/4(Delta)
  [Pos] -> Subsystem13/2(Pos)
  [PosTolr] -> Subsystem13/5(Tolr)
  [PosV] -> Subsystem13/1(PosV)
  Subsystem13/2(IsPosZone) -> [Md61IsTargetPosZone]
  Subsystem13/3(IsPosAlready) -> [Md61IsTargetPosAlready]
  Subsystem13/1(IsPos) -> [Md61IsTargetPos]
  Subsystem14/1(IsPos) -> [Md62IsTargetPos]
  Subsystem14/3(IsPosAlready) -> [Md62IsTargetPosAlready]
  Subsystem14/2(IsPosZone) -> [Md62IsTargetPosZone]
  [PosV] -> Subsystem14/1(PosV)
  [PosTolr] -> Subsystem14/5(Tolr)
  [Pos] -> Subsystem14/2(Pos)
  [PosDelta] -> Subsystem14/4(Delta)
  [Md62Calib] -> Subsystem14/3(CalibArray)
  [Md61Calib] -> Subsystem/13(Md61Calib)
  [Md62Calib] -> Subsystem/14(Md62Calib)
  [Md61IsTargetPos] -> Subsystem1/34(Md61IsTargetPos)
  [Md62IsTargetPos] -> Subsystem1/35(Md62IsTargetPos)
  [Md61IsTargetPosAlready] -> Subsystem1/36(Md61IsTargetPosAlready)
  [Md62IsTargetPosAlready] -> Subsystem1/37(Md62IsTargetPosAlready)
  [Md61IsTargetPosZone] -> Subsystem1/38(Md61IsTargetPosZone)
  [Md62IsTargetPosZone] -> Subsystem1/39(Md62IsTargetPosZone)
  VIPLExitR3LFwdBkwdTrgtPosCalib_TrgtPosArray_read/1 -> [Md27Calib]
  Md27R3LFwdBkwdTrgtPosCalib_TrgtPosArray_read/1 -> [Md14Calib]
  [Md14Calib] -> Subsystem3/3(CalibArray)

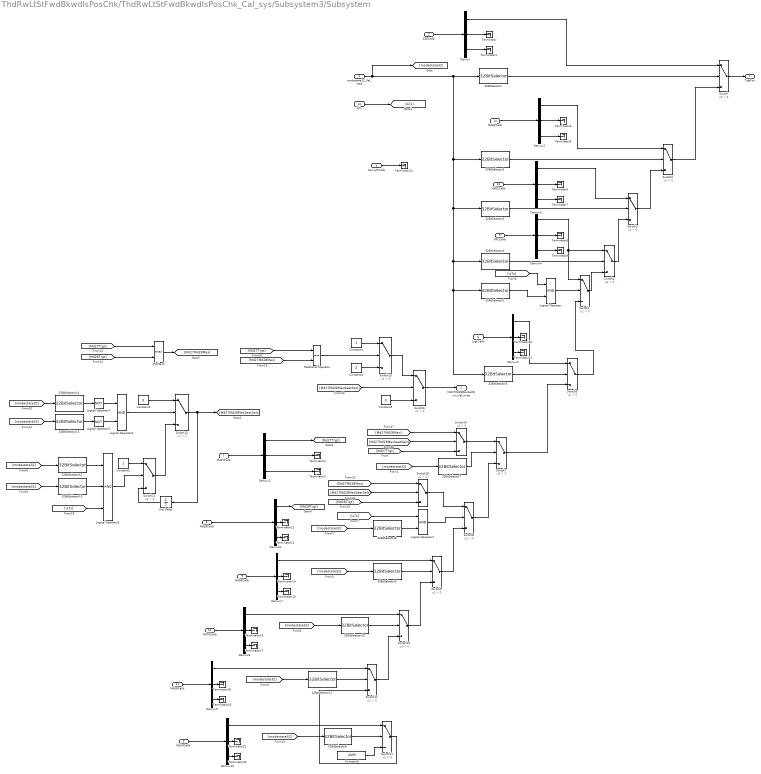
== system ThdRwLtStFwdBkwdIsPosChk/ThdRwLtStFwdBkwdIsPosChk_Cal_sys/Subsystem3/Subsystem ==
  modestate32_Val_read : Inport
  EZECalib : Inport  Port=2
  Md14Calib : Inport  Port=3
  FamlyRCalib : Inport  Port=4
  VIPLCalib : Inport  Port=5
  LugLCalib : Inport  Port=6
  Md27Calib : Inport  Port=7
  Md28Calib : Inport  Port=8
  Md56Calib : Inport  Port=9
  Md76Calib : Inport  Port=10
  Md58Calib : Inport  Port=11
  is7s : Inport  Port=12
  Md61Calib : Inport  Port=13
  Md62Calib : Inport  Port=14
  32BitSelector : StIsPosChkLib/32BitSelector  BitNum=0  SSRTWFcnClass=[]
  32BitSelector1 : StIsPosChkLib/32BitSelector  BitNum=11  SSRTWFcnClass=[]
  32BitSelector10 : StIsPosChkLib/32BitSelector  BitNum=20  SSRTWFcnClass=[]
  32BitSelector11 : StIsPosChkLib/32BitSelector  BitNum=21  SSRTWFcnClass=[]
  32BitSelector12 : StIsPosChkLib/32BitSelector  BitNum=26  SSRTWFcnClass=[]
  32BitSelector13 : StIsPosChkLib/32BitSelector  BitNum=27  SSRTWFcnClass=[]
  32BitSelector14 : StIsPosChkLib/32BitSelector  BitNum=26  SSRTWFcnClass=[]
  32BitSelector15 : StIsPosChkLib/32BitSelector  BitNum=27  SSRTWFcnClass=[]
  32BitSelector2 : StIsPosChkLib/32BitSelector  BitNum=6  SSRTWFcnClass=[]
  32BitSelector3 : StIsPosChkLib/32BitSelector  BitNum=5  SSRTWFcnClass=[]
  32BitSelector4 : StIsPosChkLib/32BitSelector  BitNum=9  SSRTWFcnClass=[]
  32BitSelector5 : StIsPosChkLib/32BitSelector  BitNum=7  SSRTWFcnClass=[]
  32BitSelector6 : StIsPosChkLib/32BitSelector  BitNum=13  SSRTWFcnClass=[]
  32BitSelector7 : StIsPosChkLib/32BitSelector  BitNum=26  SSRTWFcnClass=[]
  32BitSelector8 : StIsPosChkLib/32BitSelector  BitNum=27  SSRTWFcnClass=[]
  32BitSelector9 : StIsPosChkLib/32BitSelector  BitNum=24  SSRTWFcnClass=[]
  Constant1 : Constant  Value=0  OutDataTypeStr=boolean
  Constant2 : Constant  OutDataTypeStr=boolean
  Constant3 : Constant  OutDataTypeStr=uint8
  Constant4 : Constant  Value=2  OutDataTypeStr=uint8
  Constant5 : Constant  Value=0  OutDataTypeStr=uint8
  Constant6 : Constant  Value=4095  OutDataTypeStr=uint16
  Demux{,1..10} (11 alike) : Demux  Outputs=3
  Logical Operator : Logic  AllPortsSameDT=off  OutDataTypeStr=boolean
  Logical Operator1 : Logic  AllPortsSameDT=off  OutDataTypeStr=boolean
  Logical Operator2 : Logic  Inputs=3  AllPortsSameDT=off  OutDataTypeStr=boolean
  Logical Operator3 : Logic  AllPortsSameDT=off  OutDataTypeStr=boolean
  Logical Operator4 : Logic  Operator=NOT  AllPortsSameDT=off  OutDataTypeStr=boolean
  Logical Operator5 : Logic  Operator=NOT  AllPortsSameDT=off  OutDataTypeStr=boolean
  MinMax1 : MinMax  Function=max  Inputs=2
  Relational Operator : RelationalOperator  Operator===  OutDataTypeStr=boolean  RndMeth=Simplest
  Switch{,1..17} (18 alike) : Switch  Criteria=u2 > Threshold
  Terminator{,1..19,21..23} (23 alike) : Terminator
  Unit Delay : UnitDelay  SampleTime=-1
  TrgtPos : Outport
      settings: EnsureOutportIsVirtual=on
  Md27Md28MaxSelcNum_Val_write : Outport  Port=2
      settings: EnsureOutportIsVirtual=on
  wires:
  32BitSelector/1 -> Switch/2
  Demux/1 -> Switch/1
  Demux/3 -> Terminator1/1
  Demux/2 -> Terminator/1
  EZECalib/1 -> Demux/1
  Switch/1 -> TrgtPos/1
  Switch2/1 -> Switch/3
  Switch3/1 -> Switch2/3
  Switch4/1 -> Switch3/3
  32BitSelector2/1 -> Switch2/2
  32BitSelector3/1 -> Switch3/2
  32BitSelector4/1 -> Switch4/2
  Demux2/1 -> Switch2/1
  Demux2/3 -> Terminator5/1
  Demux2/2 -> Terminator4/1
  Demux3/2 -> Terminator6/1
  Demux3/3 -> Terminator7/1
  Demux3/1 -> Switch3/1
  Demux4/1 -> Switch4/1, Switch1/1
  Demux4/3 -> Terminator9/1
  Demux4/2 -> Terminator8/1
  VIPLCalib/1 -> Demux4/1
  LugLCalib/1 -> Demux5/1
  Demux5/2 -> Terminator10/1
  Demux5/3 -> Terminator11/1
  Demux5/1 -> Switch5/1
  32BitSelector5/1 -> Switch5/2
  Switch1/1 -> Switch4/3
  Switch5/1 -> Switch1/3
  Demux1/1 -> [Md27Trgt]
  Demux1/3 -> Terminator3/1
  Demux1/2 -> Terminator2/1
  Md27Calib/1 -> Demux1/1
  Md28Calib/1 -> Demux6/1
  Demux6/2 -> Terminator12/1
  Demux6/3 -> Terminator13/1
  modestate32_Val_read/1 -> [modestate32], 32BitSelector2/1, 32BitSelector1/1, 32BitSelector5/1, 32BitSelector4/1, 32BitSelector3/1, 32BitSelector/1
  Switch7/1 -> Switch5/3
  Switch8/1 -> Switch7/3
  32BitSelector7/1 -> Switch7/2
  [modestate32] -> 32BitSelector7/1
  [modestate32] -> 32BitSelector8/1
  Switch9/1 -> Switch8/3
  Demux7/1 -> Switch9/1
  Demux7/3 -> Terminator15/1
  Demux7/2 -> Terminator14/1
  Md56Calib/1 -> Demux7/1
  32BitSelector9/1 -> Switch9/2
  [modestate32] -> 32BitSelector9/1
  [modestate32] -> 32BitSelector10/1
  32BitSelector10/1 -> Switch10/2
  Switch10/1 -> Switch9/3
  Switch11/1 -> Switch10/3
  32BitSelector11/1 -> Switch11/2
  [modestate32] -> 32BitSelector11/1
  Md76Calib/1 -> Demux8/1
  Demux8/2 -> Terminator16/1
  Demux8/3 -> Terminator17/1
  Demux8/1 -> Switch10/1
  Demux9/1 -> Switch11/1
  Demux9/3 -> Terminator19/1
  Demux9/2 -> Terminator18/1
  Md58Calib/1 -> Demux9/1
  is7s/1 -> [is7s]
  Logical Operator/1 -> Switch1/2
  32BitSelector1/1 -> Logical Operator/2
  [is7s] -> Logical Operator/1
  [is7s] -> Logical Operator1/1
  32BitSelector8/1 -> Logical Operator1/2
  Logical Operator1/1 -> Switch8/2
  [modestate32] -> 32BitSelector12/1
  [modestate32] -> 32BitSelector13/1
  32BitSelector12/1 -> Logical Operator2/1
  32BitSelector13/1 -> Logical Operator2/2
  [modestate32] -> 32BitSelector14/1
  32BitSelector14/1 -> Logical Operator4/1
  32BitSelector15/1 -> Logical Operator5/1
  [modestate32] -> 32BitSelector15/1
  Logical Operator4/1 -> Logical Operator3/1
  Logical Operator5/1 -> Logical Operator3/2
  Logical Operator2/1 -> Switch12/2
  Logical Operator3/1 -> Switch13/2
  Constant1/1 -> Switch13/1
  Constant2/1 -> Switch12/1
  Switch12/1 -> Switch13/3
  Switch13/1 -> Unit Delay/1, [Md27Md28MaxSeatSelc]
  Unit Delay/1 -> Switch12/3
  [Md27Trgt] -> MinMax1/1
  [Md28Trgt] -> MinMax1/2
  MinMax1/1 -> [Md27Md28Max]
  Switch14/1 -> Switch7/1
  [Md27Md28MaxSeatSelc] -> Switch14/2
  [Md27Md28Max] -> Switch14/1
  [Md27Trgt] -> Switch14/3
  Demux6/1 -> [Md28Trgt]
  [is7s] -> Logical Operator2/3
  [Md27Md28Max] -> Relational Operator/2
  [Md27Trgt] -> Relational Operator/1
  [Md27Md28MaxSeatSelc] -> Switch6/2
  Relational Operator/1 -> Switch15/2
  Constant3/1 -> Switch15/1
  Constant4/1 -> Switch15/3
  Constant5/1 -> Switch6/3
  Switch15/1 -> Switch6/1
  Switch6/1 -> Md27Md28MaxSelcNum_Val_write/1
  Switch16/1 -> Switch8/1
  [Md28Trgt] -> Switch16/3
  [Md27Md28Max] -> Switch16/1
  [Md27Md28MaxSeatSelc] -> Switch16/2
  Md61Calib/1 -> Demux3/1
  Md62Calib/1 -> Demux2/1
  FamlyRCalib/1 -> Terminator21/1
  Demux10/1 -> Switch17/1
  Constant6/1 -> Switch17/3
  [modestate32] -> 32BitSelector6/1
  Demux10/2 -> Terminator22/1
  32BitSelector6/1 -> Switch17/2
  Demux10/3 -> Terminator23/1
  Md14Calib/1 -> Demux10/1
  Switch17/1 -> Switch11/3

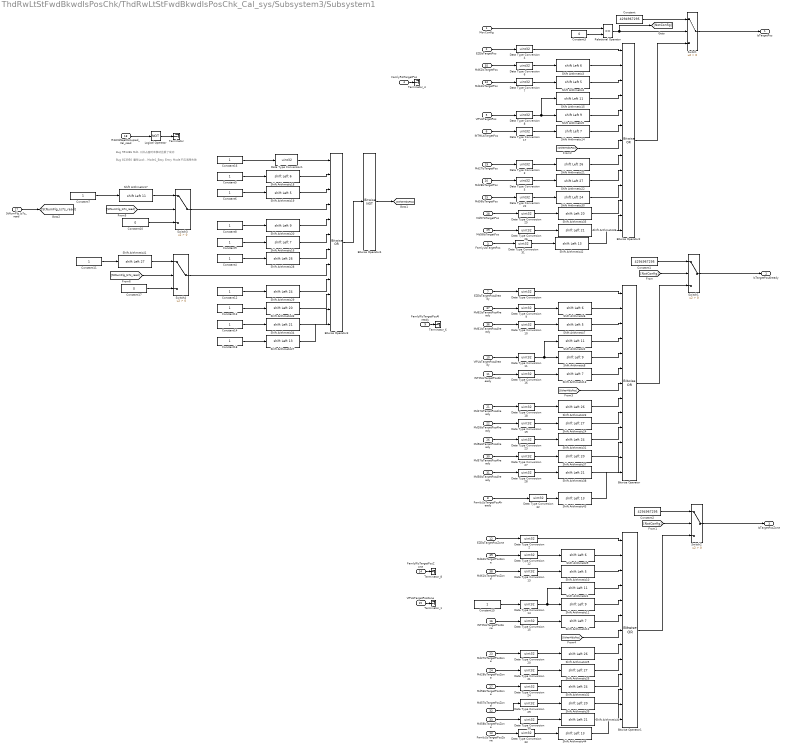
== system ThdRwLtStFwdBkwdIsPosChk/ThdRwLtStFwdBkwdIsPosChk_Cal_sys/Subsystem3/Subsystem1 ==
  note: Bug 991386 Md1 三排占座时未移动且报了成功
  note: Bug 813950 童锁Lock，Mode1_Easy Entry Mode 不应调用失败
  MovConfig : Inport
  EZEIsTargetPos : Inport  Port=2
  FamlyLIsTargetPos : Inport  Port=3
  FamlyRIsTargetPos : Inport  Port=4
  VIPLIsTargetPos : Inport  Port=5
  INTMLIsTargetPos : Inport  Port=6
  EZEIsTargetPosAlready : Inport  Port=7
  FamlyLIsTargetPosAlready : Inport  Port=8
  FamlyRIsTargetPosAlready : Inport  Port=9
  VIPLIsTargetPosAlready : Inport  Port=10
  INTMLIsTargetPosAlready : Inport  Port=11
  EZEIsTargetPosZone : Inport  Port=12
  FamlyLIsTargetPosZone : Inport  Port=13
  FamlyRIsTargetPosZone : Inport  Port=14
  VIPLIsTargetPosZone : Inport  Port=15
  INTMLIsTargetPosZone : Inport  Port=16
  StNumFlg_Is7s_read : Inport  Port=17
  R3LMdSeatOccupied_Val_read : Inport  Port=18
  Md27IsTargetPos : Inport  Port=19
  Md28IsTargetPos : Inport  Port=20
  Md27IsTargetPosAlready : Inport  Port=21
  Md28IsTargetPosAlready : Inport  Port=22
  Md27IsTargetPosZone : Inport  Port=23
  Md28IsTargetPosZone : Inport  Port=24
  Md56IsTargetPos : Inport  Port=25
  Md56IsTargetPosAlready : Inport  Port=26
  Md56IsTargetPosZone : Inport  Port=27
  Md57IsTargetPos : Inport  Port=28
  Md58IsTargetPos : Inport  Port=29
  Md57IsTargetPosAlready : Inport  Port=30
  Md58IsTargetPosAlready : Inport  Port=31
  Md57IsTargetPosZone : Inport  Port=32
  Md58IsTargetPosZone : Inport  Port=33
  Md61IsTargetPos : Inport  Port=34
  Md62IsTargetPos : Inport  Port=35
  Md61IsTargetPosAlready : Inport  Port=36
  Md62IsTargetPosAlready : Inport  Port=37
  Md61IsTargetPosZone : Inport  Port=38
  Md62IsTargetPosZone : Inport  Port=39
  Bitwise Operator : simulink/Logic and Bit Operations/Bitwise Operator  logicop=OR  UseBitMask=off  NumInputPorts=13  BitMask=bin2dec('11011001')  BitMaskRealWorld=Stored Integer
  Bitwise Operator1 : simulink/Logic and Bit Operations/Bitwise Operator  logicop=OR  UseBitMask=off  NumInputPorts=13  BitMask=bin2dec('11011001')  BitMaskRealWorld=Stored Integer
  Bitwise Operator2 : simulink/Logic and Bit Operations/Bitwise Operator  logicop=OR  UseBitMask=off  NumInputPorts=13  BitMask=bin2dec('11011001')  BitMaskRealWorld=Stored Integer
  Bitwise Operator3 : simulink/Logic and Bit Operations/Bitwise Operator  logicop=OR  UseBitMask=off  NumInputPorts=12  BitMask=bin2dec('11011001')  BitMaskRealWorld=Stored Integer
  Bitwise Operator4 : simulink/Logic and Bit Operations/Bitwise Operator  logicop=NOT  UseBitMask=off  BitMask=bin2dec('11011001')  BitMaskRealWorld=Stored Integer
  Constant : Constant  Value=4294967295  OutDataTypeStr=uint32
  Constant1 : Constant  Value=4294967295  OutDataTypeStr=uint32
  Constant10 : Constant  Value=0  OutDataTypeStr=uint32
  Constant{4..9,11..16,18} (13 alike) : Constant  OutDataTypeStr=uint32
  Constant17 : Constant  Value=0  OutDataTypeStr=uint32
  Constant2 : Constant  Value=4294967295  OutDataTypeStr=uint32
  Constant3 : Constant  Value=0  OutDataTypeStr=uint8
  Data Type Conversion{,1..33} (34 alike) : DataTypeConversion  OutDataTypeStr=uint32
  Logical Operator : Logic  Operator=NOT  AllPortsSameDT=off  OutDataTypeStr=boolean
  Relational Operator : RelationalOperator  Operator===  OutDataTypeStr=boolean  RndMeth=Simplest
  Shift Arithmetic{1..2,15,17} (4 alike) : ArithShift  BitShiftNumber=11  BitShiftDirection=Left
  Shift Arithmetic{4,7,10,19} (4 alike) : ArithShift  BitShiftNumber=5  BitShiftDirection=Left
  Shift Arithmetic{5,8,11,20} (4 alike) : ArithShift  BitShiftNumber=9  BitShiftDirection=Left
  Shift Arithmetic{12..14,16} (4 alike) : ArithShift  BitShiftNumber=7  BitShiftDirection=Left
  Shift Arithmetic{3,6,9,18} (4 alike) : ArithShift  BitShiftNumber=6  BitShiftDirection=Left
  Shift Arithmetic{21,23,25,28} (4 alike) : ArithShift  BitShiftNumber=26  BitShiftDirection=Left
  Shift Arithmetic{22,24,26,41} (4 alike) : ArithShift  BitShiftNumber=27  BitShiftDirection=Left
  Shift Arithmetic{27,42..44} (4 alike) : ArithShift  BitShiftNumber=13  BitShiftDirection=Left
  Shift Arithmetic{29..32} (4 alike) : ArithShift  BitShiftNumber=24  BitShiftDirection=Left
  Shift Arithmetic{33,35,37,39} (4 alike) : ArithShift  BitShiftNumber=20  BitShiftDirection=Left
  Shift Arithmetic{34,36,38,40} (4 alike) : ArithShift  BitShiftNumber=21  BitShiftDirection=Left
  Switch{,1..4} (5 alike) : Switch  Criteria=u2 > Threshold
  Terminator : Terminator
  Terminator_{1,4,6,8} (4 alike) : Terminator
  IsTargetPos : Outport
      settings: EnsureOutportIsVirtual=on
  IsTargetPosAlready : Outport  Port=2
      settings: EnsureOutportIsVirtual=on
  IsTargetPosZone : Outport  Port=3
      settings: EnsureOutportIsVirtual=on
  wires:
  Constant3/1 -> Relational Operator/2
  Constant/1 -> Switch/1
  Relational Operator/1 -> [NotConfig], Switch/2
  MovConfig/1 -> Relational Operator/1
  Switch/1 -> IsTargetPos/1
  [NotConfig] -> Switch1/2
  Constant1/1 -> Switch1/1
  Switch1/1 -> IsTargetPosAlready/1
  Switch2/1 -> IsTargetPosZone/1
  Constant2/1 -> Switch2/1
  [NotConfig] -> Switch2/2
  Data Type Conversion/1 -> Bitwise Operator/1
  Data Type Conversion2/1 -> Bitwise Operator1/1
  Bitwise Operator1/1 -> Switch2/3
  Bitwise Operator/1 -> Switch1/3
  Data Type Conversion4/1 -> Bitwise Operator2/1
  Bitwise Operator2/1 -> Switch/3
  EZEIsTargetPos/1 -> Data Type Conversion4/1
  EZEIsTargetPosZone/1 -> Data Type Conversion2/1
  EZEIsTargetPosAlready/1 -> Data Type Conversion/1
  Shift Arithmetic3/1 -> Bitwise Operator2/2
  Shift Arithmetic4/1 -> Bitwise Operator2/3
  Shift Arithmetic5/1 -> Bitwise Operator2/5
  Data Type Conversion7/1 -> Shift Arithmetic4/1
  Data Type Conversion6/1 -> Shift Arithmetic3/1
  Data Type Conversion8/1 -> Shift Arithmetic15/1, Shift Arithmetic5/1
  VIPLIsTargetPos/1 -> Data Type Conversion8/1
  VIPLIsTargetPosAlready/1 -> Data Type Conversion11/1
  Data Type Conversion11/1 -> Shift Arithmetic2/1, Shift Arithmetic8/1
  Data Type Conversion9/1 -> Shift Arithmetic6/1
  Data Type Conversion10/1 -> Shift Arithmetic7/1
  Shift Arithmetic8/1 -> Bitwise Operator/5
  Shift Arithmetic7/1 -> Bitwise Operator/3
  Shift Arithmetic6/1 -> Bitwise Operator/2
  Data Type Conversion14/1 -> Shift Arithmetic1/1, Shift Arithmetic11/1
  Data Type Conversion13/1 -> Shift Arithmetic10/1
  Shift Arithmetic10/1 -> Bitwise Operator1/3
  Shift Arithmetic9/1 -> Bitwise Operator1/2
  Shift Arithmetic11/1 -> Bitwise Operator1/5
  Data Type Conversion12/1 -> Shift Arithmetic9/1
  Shift Arithmetic12/1 -> Bitwise Operator1/6
  Data Type Conversion15/1 -> Shift Arithmetic12/1
  INTMLIsTargetPosZone/1 -> Data Type Conversion15/1
  Shift Arithmetic13/1 -> Bitwise Operator/6
  Data Type Conversion16/1 -> Shift Arithmetic13/1
  INTMLIsTargetPosAlready/1 -> Data Type Conversion16/1
  Shift Arithmetic14/1 -> Bitwise Operator2/6
  Data Type Conversion17/1 -> Shift Arithmetic14/1
  INTMLIsTargetPos/1 -> Data Type Conversion17/1
  Shift Arithmetic1/1 -> Bitwise Operator1/4
  Shift Arithmetic2/1 -> Bitwise Operator/4
  Shift Arithmetic15/1 -> Bitwise Operator2/4
  Shift Arithmetic16/1 -> Bitwise Operator3/6
  Shift Arithmetic20/1 -> Bitwise Operator3/5
  Shift Arithmetic19/1 -> Bitwise Operator3/3
  Shift Arithmetic18/1 -> Bitwise Operator3/2
  Data Type Conversion1/1 -> Bitwise Operator3/1
  Constant5/1 -> Shift Arithmetic18/1
  Constant6/1 -> Shift Arithmetic19/1
  Constant7/1 -> Shift Arithmetic17/1
  Constant8/1 -> Shift Arithmetic20/1
  Constant9/1 -> Shift Arithmetic16/1
  Bitwise Operator3/1 -> Bitwise Operator4/1
  Bitwise Operator4/1 -> [OtherMdIsPos]
  [OtherMdIsPos] -> Bitwise Operator2/7
  [OtherMdIsPos] -> Bitwise Operator/7
  [OtherMdIsPos] -> Bitwise Operator1/7
  Shift Arithmetic17/1 -> Switch3/1
  Switch3/1 -> Bitwise Operator3/4
  Constant10/1 -> Switch3/3
  R3LMdSeatOccupied_Val_read/1 -> Logical Operator/1
  Md27IsTargetPos/1 -> Data Type Conversion3/1
  Md28IsTargetPos/1 -> Data Type Conversion5/1
  Data Type Conversion3/1 -> Shift Arithmetic21/1
  Shift Arithmetic21/1 -> Bitwise Operator2/8
  Shift Arithmetic22/1 -> Bitwise Operator2/9
  Data Type Conversion5/1 -> Shift Arithmetic22/1
  Md28IsTargetPosAlready/1 -> Data Type Conversion19/1
  Md27IsTargetPosAlready/1 -> Data Type Conversion18/1
  Md27IsTargetPosZone/1 -> Data Type Conversion20/1
  Md28IsTargetPosZone/1 -> Data Type Conversion21/1
  Data Type Conversion18/1 -> Shift Arithmetic23/1
  Data Type Conversion19/1 -> Shift Arithmetic24/1
  Data Type Conversion20/1 -> Shift Arithmetic25/1
  Data Type Conversion21/1 -> Shift Arithmetic26/1
  Shift Arithmetic25/1 -> Bitwise Operator1/8
  Shift Arithmetic23/1 -> Bitwise Operator/8
  Shift Arithmetic24/1 -> Bitwise Operator/9
  Shift Arithmetic26/1 -> Bitwise Operator1/9
  Constant4/1 -> Shift Arithmetic28/1
  Shift Arithmetic28/1 -> Bitwise Operator3/7
  Switch4/1 -> Bitwise Operator3/8
  Constant12/1 -> Shift Arithmetic29/1
  Shift Arithmetic29/1 -> Bitwise Operator3/9
  Data Type Conversion22/1 -> Shift Arithmetic30/1
  Shift Arithmetic30/1 -> Bitwise Operator2/10
  Md56IsTargetPos/1 -> Data Type Conversion22/1
  Shift Arithmetic31/1 -> Bitwise Operator/10
  Data Type Conversion23/1 -> Shift Arithmetic31/1
  Md56IsTargetPosAlready/1 -> Data Type Conversion23/1
  Shift Arithmetic32/1 -> Bitwise Operator1/10
  Data Type Conversion24/1 -> Shift Arithmetic32/1
  Md56IsTargetPosZone/1 -> Data Type Conversion24/1
  Shift Arithmetic33/1 -> Bitwise Operator3/10
  Constant13/1 -> Shift Arithmetic33/1
  Constant14/1 -> Shift Arithmetic34/1
  Shift Arithmetic34/1 -> Bitwise Operator3/11
  Md57IsTargetPos/1 -> Data Type Conversion25/1
  Shift Arithmetic35/1 -> Bitwise Operator2/11
  Data Type Conversion25/1 -> Shift Arithmetic35/1
  Data Type Conversion26/1 -> Shift Arithmetic36/1
  Shift Arithmetic36/1 -> Bitwise Operator2/12
  Md58IsTargetPos/1 -> Data Type Conversion26/1
  Md57IsTargetPosAlready/1 -> Data Type Conversion27/1
  Data Type Conversion27/1 -> Shift Arithmetic37/1
  Shift Arithmetic37/1 -> Bitwise Operator/11
  Shift Arithmetic38/1 -> Bitwise Operator/12
  Data Type Conversion28/1 -> Shift Arithmetic38/1
  Md58IsTargetPosAlready/1 -> Data Type Conversion28/1
  Md57IsTargetPosZone/1 -> Data Type Conversion29/1
  Data Type Conversion29/1 -> Shift Arithmetic39/1
  Shift Arithmetic39/1 -> Bitwise Operator1/11
  Shift Arithmetic40/1 -> Bitwise Operator1/12
  Data Type Conversion30/1 -> Shift Arithmetic40/1
  Md58IsTargetPosZone/1 -> Data Type Conversion30/1
  Constant15/1 -> Data Type Conversion14/1
  VIPLIsTargetPosZone/1 -> Terminator_1/1
  Constant16/1 -> Data Type Conversion1/1
  Logical Operator/1 -> Terminator/1
  Md61IsTargetPosZone/1 -> Data Type Conversion13/1
  Md62IsTargetPosZone/1 -> Data Type Conversion12/1
  Md62IsTargetPosAlready/1 -> Data Type Conversion9/1
  Md61IsTargetPosAlready/1 -> Data Type Conversion10/1
  Md62IsTargetPos/1 -> Data Type Conversion6/1
  Md61IsTargetPos/1 -> Data Type Conversion7/1
  StNumFlg_Is7s_read/1 -> [StNumFlg_Is7s_read]
  [StNumFlg_Is7s_read] -> Switch3/2
  Constant17/1 -> Switch4/3
  Shift Arithmetic41/1 -> Switch4/1
  Constant11/1 -> Shift Arithmetic41/1
  [StNumFlg_Is7s_read] -> Switch4/2
  FamlyRIsTargetPos/1 -> Terminator_4/1
  FamlyLIsTargetPosAlready/1 -> Data Type Conversion32/1
  FamlyRIsTargetPosAlready/1 -> Terminator_6/1
  FamlyLIsTargetPosZone/1 -> Data Type Conversion33/1
  FamlyRIsTargetPosZone/1 -> Terminator_8/1
  Constant18/1 -> Shift Arithmetic27/1
  Shift Arithmetic27/1 -> Bitwise Operator3/12
  Data Type Conversion31/1 -> Shift Arithmetic42/1
  FamlyLIsTargetPos/1 -> Data Type Conversion31/1
  Shift Arithmetic42/1 -> Bitwise Operator2/13
  Data Type Conversion32/1 -> Shift Arithmetic43/1
  Shift Arithmetic43/1 -> Bitwise Operator/13
  Data Type Conversion33/1 -> Shift Arithmetic44/1
  Shift Arithmetic44/1 -> Bitwise Operator1/13

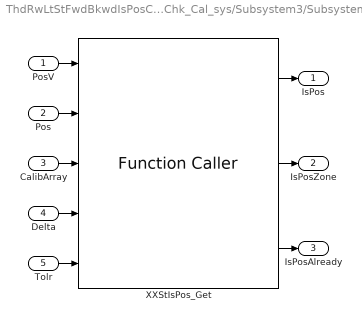
== system ThdRwLtStFwdBkwdIsPosChk/ThdRwLtStFwdBkwdIsPosChk_Cal_sys/Subsystem3/Subsystem10 ==
  PosV : Inport
  Pos : Inport  Port=2
  CalibArray : Inport  Port=3
  Delta : Inport  Port=4
  Tolr : Inport  Port=5
  XXStIsPos_Get : FunctionCaller  FunctionPrototype=[IsPos,IsPosZone,IsPosAlready] = XXStIsPos_Get(PosV,Pos,CalibArray,Delta,Tolr)  InputArgumentSpecifications=boolean(true), uint16(1), uint16([1;1;1]), uint16(1), uint16(1)  OutputArgumentSpecifications=boolean(true), boolean(true), boolean(true)
  IsPos : Outport
  IsPosZone : Outport  Port=2
  IsPosAlready : Outport  Port=3
  wires:
  Pos/1 -> XXStIsPos_Get/2
  Delta/1 -> XXStIsPos_Get/4
  CalibArray/1 -> XXStIsPos_Get/3
  XXStIsPos_Get/2 -> IsPosZone/1
  XXStIsPos_Get/1 -> IsPos/1
  Tolr/1 -> XXStIsPos_Get/5
  XXStIsPos_Get/3 -> IsPosAlready/1
  PosV/1 -> XXStIsPos_Get/1

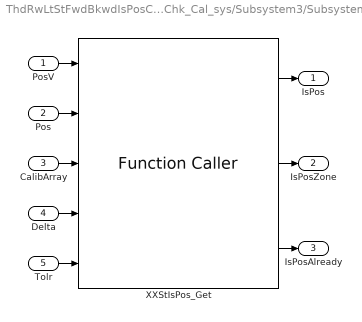
== system ThdRwLtStFwdBkwdIsPosChk/ThdRwLtStFwdBkwdIsPosChk_Cal_sys/Subsystem3/Subsystem11 ==
  PosV : Inport
  Pos : Inport  Port=2
  CalibArray : Inport  Port=3
  Delta : Inport  Port=4
  Tolr : Inport  Port=5
  XXStIsPos_Get : FunctionCaller  FunctionPrototype=[IsPos,IsPosZone,IsPosAlready] = XXStIsPos_Get(PosV,Pos,CalibArray,Delta,Tolr)  InputArgumentSpecifications=boolean(true), uint16(1), uint16([1;1;1]), uint16(1), uint16(1)  OutputArgumentSpecifications=boolean(true), boolean(true), boolean(true)
  IsPos : Outport
  IsPosZone : Outport  Port=2
  IsPosAlready : Outport  Port=3
  wires:
  PosV/1 -> XXStIsPos_Get/1
  XXStIsPos_Get/3 -> IsPosAlready/1
  Tolr/1 -> XXStIsPos_Get/5
  XXStIsPos_Get/1 -> IsPos/1
  XXStIsPos_Get/2 -> IsPosZone/1
  CalibArray/1 -> XXStIsPos_Get/3
  Delta/1 -> XXStIsPos_Get/4
  Pos/1 -> XXStIsPos_Get/2
